simulink library "calculateReelInRudderAngle"  (R2018a)
settings: Solver=VariableStepAuto  StartTime=0.0  StopTime=10.0  RelTol=1e-3
undefined symbols (not defined in the file): ctrl
settings Model: Creator=mitch  LastModifiedBy=mitch

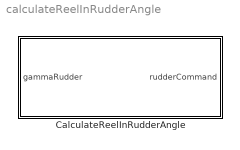
== system calculateReelInRudderAngle ==
  CalculateReelInRudderAngle : Subsystem

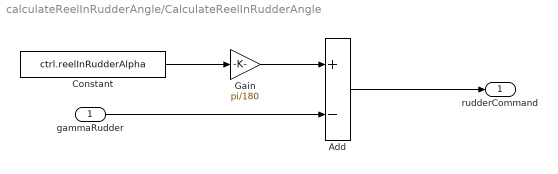
== system calculateReelInRudderAngle/CalculateReelInRudderAngle ==
  gammaRudder : Inport  OutDataTypeStr=double
  Add : Sum  Inputs=+-
  Constant : Constant  Value=ctrl.reelInRudderAlpha
  Gain : Gain  Gain=pi/180
  rudderCommand : Outport
  wires:
  Add/1 -> rudderCommand/1
  Constant/1 -> Gain/1
  Gain/1 -> Add/1
  gammaRudder/1 -> Add/2
